simulink model "inverter_hil"  (R2024b)
settings: Solver=FixedStepDiscrete  StartTime=0.0  StopTime=inf  FixedStep=0.001  RelTol=1e-3
InitFcn:
  | inverterhil.enforceHardwarePreflight(bdroot);
values from neighbouring files (symbols this model uses):
  hil_cal_pedals_pressed_v1 = 1.1631952391851683    [inverter_hil.sldd]
  hil_cal_pedals_pressed_v2 = 2.341496910048066    [inverter_hil.sldd]
  hil_cal_pedals_pressed_v3 = 1.6012817578393226    [inverter_hil.sldd]
  hil_cal_pedals_pressed_v4 = 1.6012817578393226    [inverter_hil.sldd]
  hil_cal_pedals_released_v1 = 1.5156786449988555    [inverter_hil.sldd]
  hil_cal_pedals_released_v2 = 3.2025635156786452    [inverter_hil.sldd]
  hil_cal_pedals_released_v3 = 0.45445181963836118    [inverter_hil.sldd]
  hil_cal_pedals_released_v4 = 0.45445181963836118    [inverter_hil.sldd]
  hil_cmd_can_drop_control_mask = 0    [inverter_hil.sldd]
  hil_cmd_can_drop_status_mask = 0    [inverter_hil.sldd]
  hil_cmd_dc_link12_v = 0.0    [inverter_hil.sldd]
  hil_cmd_dc_link34_v = 0.0    [inverter_hil.sldd]
  hil_cmd_digital_cooling_switch = 0    [inverter_hil.sldd]
  hil_cmd_digital_main_button = 0    [inverter_hil.sldd]
  hil_cmd_digital_main_button_sequence = 0    [inverter_hil.sldd]
  hil_cmd_digital_precharge_sequence = 0    [inverter_hil.sldd]
  hil_cmd_digital_shutdown_feedback = 0    [inverter_hil.sldd]
  hil_cmd_gui_heartbeat = 0    [inverter_hil.sldd]
  hil_cmd_inverter1_connected = 1    [inverter_hil.sldd]
  hil_cmd_inverter1_fault_mask = 0    [inverter_hil.sldd]
  hil_cmd_inverter1_load_nm = 0.0    [inverter_hil.sldd]
  hil_cmd_inverter2_connected = 1    [inverter_hil.sldd]
  hil_cmd_inverter2_fault_mask = 0    [inverter_hil.sldd]
  hil_cmd_inverter2_load_nm = 0.0    [inverter_hil.sldd]
  hil_cmd_inverter3_connected = 1    [inverter_hil.sldd]
  hil_cmd_inverter3_fault_mask = 0    [inverter_hil.sldd]
  hil_cmd_inverter3_load_nm = 0.0    [inverter_hil.sldd]
  hil_cmd_inverter4_connected = 1    [inverter_hil.sldd]
  hil_cmd_inverter4_fault_mask = 0    [inverter_hil.sldd]
  hil_cmd_inverter4_load_nm = 0.0    [inverter_hil.sldd]
  hil_cmd_pedals_brake = 0.0    [inverter_hil.sldd]
  hil_cmd_pedals_plausibility_override = 0    [inverter_hil.sldd]
  hil_cmd_pedals_throttle = 0.0    [inverter_hil.sldd]
undefined symbols (not defined in the file or in its folder): Pull, up
libraries: speedgoatlib_IO614 x18, canmsglib x14, speedgoatlib_IO183 x8
(part 2 of 2)

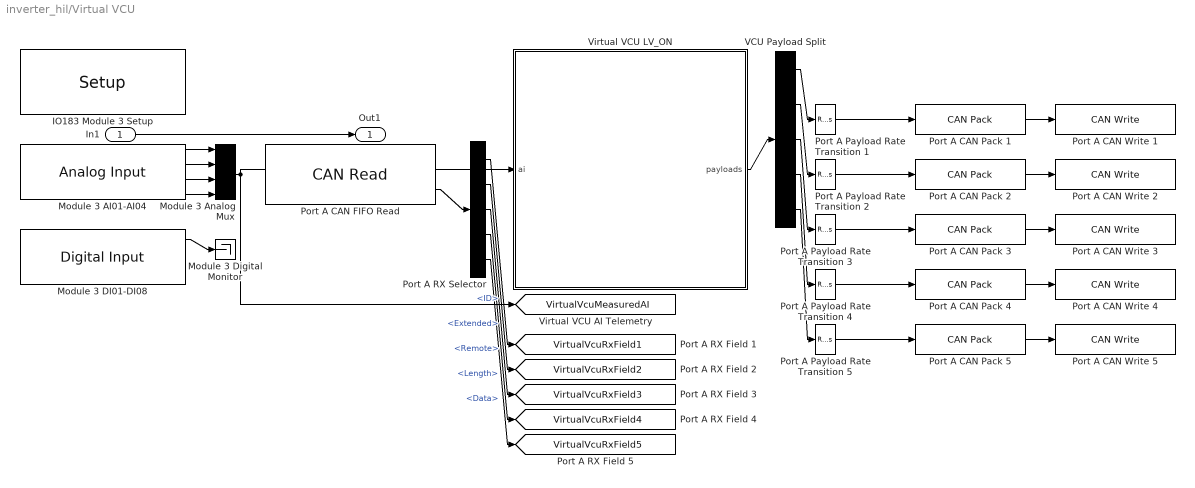
== system inverter_hil/Virtual VCU ==
  In1 : Inport
  IO183 Module 3 Setup : speedgoatlib_IO183/Setup  parModuleId=3  parPciSlot=-1  parDaSimult=on  parAdCoupling=Single Ended  parAdRange=0..5V  parAdChannelLow=1  parAdChannelHigh=4  parDaChannels=[1 2 3 4]  parDaRange=0..5V  parDaInit=[0 0 0 0]  parDaReset=[0 0 0 0]  parDoChannels=[1 2 3 4 5 6 7 8]  parDoInit=[0 0 0 0 0 0 0 0]  parDoReset=[0 0 0 0 0 0 0 0]  parDiChannels=[1 2 3 4 5 6 7 8]  parIOPullReferenceFront=Pull-down  parIOPullReferenceRear=Pull-up (3.3V)
      settings: SourceProductName=IO183
  Module 3 AI01-AI04 : speedgoatlib_IO183/Analog Input  Priority=0  parModuleId=3  parSampTime=0.001  parPciSlot=-1  parAdChannelLow=1  parAdChannelHigh=4
      settings: SourceProductName=IO183
  Module 3 Analog Mux : Mux
  Module 3 DI01-DI08 : speedgoatlib_IO183/Digital Input  parModuleId=3  parSampTime=0.001  parPciSlot=-1  parDiChannels=[1 2 3 4 5 6 7 8]
      settings: SourceProductName=IO183
  Module 3 Digital Monitor : Terminator
  Port A CAN FIFO Read : speedgoatlib_IO614/CAN Read   moduleType=IO614  id=1  channel=2  canType=CAN (HS)  useBusOut=on  HasMulRead=Single Read from Buffer (FIFO)  MsgIDlist=[1 2]  isEFF=off  LabelInHex=on  enableInput=off  ts=0.001  initValues=[614 1 0.001 1 1 1 0 1 0 1 2 1 2]
      settings: SourceProductName=IO614
  Port A CAN Pack 1 : canmsglib/CAN Pack  MsgList=(none)  MsgName=CAN Msg  MsgIDType=Standard (11-bit identifier)  MsgIdentifier=501  CANIDInput=off  MsgLength=8  Remote=off  ApplyMinMax=off  BusOutput=off  SignalInfo={}
      settings: LibrarySourceBlock=canlib/CAN Pack  DataFormat=raw data
  Port A CAN Pack 2 : canmsglib/CAN Pack  MsgList=(none)  MsgName=CAN Msg  MsgIDType=Standard (11-bit identifier)  MsgIdentifier=390  CANIDInput=off  MsgLength=8  Remote=off  ApplyMinMax=off  BusOutput=off  SignalInfo={}
      settings: LibrarySourceBlock=canlib/CAN Pack  DataFormat=raw data
  Port A CAN Pack 3 : canmsglib/CAN Pack  MsgList=(none)  MsgName=CAN Msg  MsgIDType=Standard (11-bit identifier)  MsgIdentifier=406  CANIDInput=off  MsgLength=8  Remote=off  ApplyMinMax=off  BusOutput=off  SignalInfo={}
      settings: LibrarySourceBlock=canlib/CAN Pack  DataFormat=raw data
  Port A CAN Pack 4 : canmsglib/CAN Pack  MsgList=(none)  MsgName=CAN Msg  MsgIDType=Standard (11-bit identifier)  MsgIdentifier=422  CANIDInput=off  MsgLength=8  Remote=off  ApplyMinMax=off  BusOutput=off  SignalInfo={}
      settings: LibrarySourceBlock=canlib/CAN Pack  DataFormat=raw data
  Port A CAN Pack 5 : canmsglib/CAN Pack  MsgList=(none)  MsgName=CAN Msg  MsgIDType=Standard (11-bit identifier)  MsgIdentifier=438  CANIDInput=off  MsgLength=8  Remote=off  ApplyMinMax=off  BusOutput=off  SignalInfo={}
      settings: LibrarySourceBlock=canlib/CAN Pack  DataFormat=raw data
  Port A CAN Write {1..5} (5 alike) : speedgoatlib_IO614/CAN Write   moduleType=IO614  id=1  channel=2  canType=CAN (HS)  useBusIn=off  numOfMsg=1  enableInput=off  enableStatusPort=on  initValues=[614 1 0.005 1 1 1 1 1 0 0]  ts=0.005
      settings: SourceProductName=IO614
  Port A Payload Rate Transition {1..5} (5 alike) : RateTransition
  Port A RX Selector : BusSelector  OutputSignals=ID,Extended,Remote,Length,Data
  VCU Payload Split : Demux  Outputs=[8 8 8 8 8]
  Virtual VCU LV_ON : MATLAB Function  TreatAsAtomicUnit=on
  Out1 : Outport
  tag scope: VirtualVcuMeasuredAI=global, VirtualVcuRxField1=global, VirtualVcuRxField2=global, VirtualVcuRxField3=global, VirtualVcuRxField4=global, VirtualVcuRxField5=global
  wires:
  In1/1 -> Out1/1
  Module 3 AI01-AI04/1 -> Module 3 Analog Mux/1
  Module 3 AI01-AI04/2 -> Module 3 Analog Mux/2
  Module 3 AI01-AI04/3 -> Module 3 Analog Mux/3
  Module 3 AI01-AI04/4 -> Module 3 Analog Mux/4
  Port A CAN FIFO Read/2 -> Port A RX Selector/1
  Module 3 Analog Mux/1 -> Virtual VCU LV_ON/1(ai), [VirtualVcuMeasuredAI]
  Virtual VCU LV_ON/1(payloads) -> VCU Payload Split/1
  Port A RX Selector/1 -> [VirtualVcuRxField1]  "<ID>"
  Port A RX Selector/2 -> [VirtualVcuRxField2]  "<Extended>"
  Port A RX Selector/3 -> [VirtualVcuRxField3]  "<Remote>"
  Port A RX Selector/4 -> [VirtualVcuRxField4]  "<Length>"
  Port A RX Selector/5 -> [VirtualVcuRxField5]  "<Data>"
  Module 3 DI01-DI08/1 -> Module 3 Digital Monitor/1
  VCU Payload Split/1 -> Port A Payload Rate Transition 1/1
  Port A Payload Rate Transition 1/1 -> Port A CAN Pack 1/1
  Port A CAN Pack 1/1 -> Port A CAN Write 1/1
  VCU Payload Split/2 -> Port A Payload Rate Transition 2/1
  Port A Payload Rate Transition 2/1 -> Port A CAN Pack 2/1
  Port A CAN Pack 2/1 -> Port A CAN Write 2/1
  VCU Payload Split/3 -> Port A Payload Rate Transition 3/1
  Port A Payload Rate Transition 3/1 -> Port A CAN Pack 3/1
  Port A CAN Pack 3/1 -> Port A CAN Write 3/1
  VCU Payload Split/4 -> Port A Payload Rate Transition 4/1
  Port A Payload Rate Transition 4/1 -> Port A CAN Pack 4/1
  Port A CAN Pack 4/1 -> Port A CAN Write 4/1
  VCU Payload Split/5 -> Port A Payload Rate Transition 5/1
  Port A Payload Rate Transition 5/1 -> Port A CAN Pack 5/1
  Port A CAN Pack 5/1 -> Port A CAN Write 5/1

== matlab function inverter_hil/Virtual VCU/Virtual VCU LV_ON ==
  data: ai input; payloads output
function payloads = virtualVcuDeployStep(ai)
%#codegen
payloads = zeros(40,1,'uint8');
t = uint8(max(0,min(100,round(ai(1) * 20))));
payloads(1) = t;
payloads(2) = uint8(max(0,min(255,round(ai(3) * 130))));
payloads(9) = 1; payloads(11) = 80; payloads(12) = 70;
payloads(17) = 1; payloads(19) = 80; payloads(20) = 70;
payloads(25) = 1; payloads(27) = 80; payloads(28) = 70;
payloads(33) = 1; payloads(35) = 80; payloads(36) = 70;
end

== matlab function inverter_hil/Hardware I O - PRE-FLIGHT DISABLED/Status Transmit Mask ==
  data: dropStatusMask input; k1 output; k2 output; k3 output; k4 output; k5 output; k6 output; k7 output; k8 output; k9 output
function [k1,k2,k3,k4,k5,k6,k7,k8,k9] = ...
    ephorusStatusTransmitMask(dropStatusMask)
%#codegen
%EPHORUSSTATUSTRANSMITMASK Fix 4: split INVERTERHIL.STATUSTRANSMITMASK's
%9-entry keep vector into nine scalar Tx Control outputs, one per
%CAN Write block in INVERTERHIL.PROTOCOL status-cycle order, because
%each CAN Write's Tx Control port takes a scalar and a MATLAB
%Function block cannot emit a bus without a Simulink.Bus definition.
%
%CAN Write's Tx Control input is uint32 (a transmit-count control, not
%a boolean enable), so KEEP is cast rather than passed as logical: 1 to
%transmit this tick, 0 to genuinely skip it.
keep = uint32(inverterhil.statusTransmitMask(dropStatusMask));
k1 = keep(1); k2 = keep(2); k3 = keep(3);
k4 = keep(4); k5 = keep(5); k6 = keep(6);
k7 = keep(7); k8 = keep(8); k9 = keep(9);
end

== matlab function inverter_hil/Ephorus System Status/Ephorus Status Cycle ==
  data: rxDataPresent input; payloads output; rxId input; rxExtended input; rxRemote input; rxLength input; rxData input; loadNm1 input; loadNm2 input; loadNm3 input; loadNm4 input; connected1 input; connected2 input; connected3 input; connected4 input; dcLink12V input; dcLink34V input; dropControlMask input; rxObservation output
function [payloads, rxObservation] = ephorusSystemStatusStep( ...
    rxDataPresent, rxId, rxExtended, rxRemote, rxLength, rxData, ...
    loadNm1, loadNm2, loadNm3, loadNm4, ...
    connected1, connected2, connected3, connected4, ...
    dcLink12V, dcLink34V, dropControlMask)
%#codegen
%EPHORUSSYSTEMSTATUSSTEP Advance the real, persistent-state Ephorus
%status cycle (see INVERTERHIL.STEPMODEL) and emit its nine 8-byte
%payloads. Single source of truth: the hardware boundary reads this
%same signal through a Goto/From pair rather than recomputing it.
%
%The RX inputs are one received CAN frame per step, published by the
%hardware boundary. BANK is persistent so a retained command survives
%across ticks, which is what lets a commanding VCU move a channel out
%of Idle.
%
%A frame is ALWAYS passed, with DROP set when nothing was received.
%RECEIVECONTROLFRAME rejects a dropped frame without touching the
%bank, so the array stays fixed-size for code generation instead of
%growing and shrinking. Nothing is fabricated: no data present means
%no command retained, exactly as before this input existed.
%
%LOADNM1-4, CONNECTED1-4, DCLINK12V/34V and DROPCONTROLMASK are GUI
%COMMAND PARAMETERS' Gotos (Fix 2, Fix 4), read here rather than by
%recomputing anything the dead "Ephorus Channel 1-4" scaffold would
%have provided.
persistent state plantState tickMs bank statusBank
if isempty(state)
    state = inverterhil.initialSystemState();
    plantState = inverterhil.initialPlantState();
    tickMs = uint32(0);
    bank = inverterhil.initialDecoderBank();
    statusBank = inverterhil.initialStatusBank();
end
%(:)' normalises the bus Data element to a 1x8 row regardless of the
%orientation Simulink propagates, matching the proven pattern in the
%IO614 CAN visibility test decoder.
payload = uint8(rxData(:))';
frame = struct( ...
    'id', uint32(rxId), ...
    'dlc', uint8(rxLength), ...
    'payload', payload, ...
    'isExtended', logical(rxExtended), ...
    'isRemote', logical(rxRemote), ...
    'drop', ~logical(rxDataPresent));
%CONFIG and CAL are passed explicitly rather than as [] so the
%variable never changes type: code generation rejects a double []
%being reassigned to a struct inside STEPMODEL's defaulting branch.
    statusBank = inverterhil.receiveStatusFrame(statusBank, frame, tickMs);
%EXTERNALINPUTS carries the GUI-commanded per-channel load torque, DC
%link pair voltage (dcLink12V feeds channels 1-2, dcLink34V feeds
%channels 3-4, matching ADDARCHITECTURE's dcPort = 1 + (channel > 2)
%convention), and connected flag into STEPMODEL -- see
%INVERTERHIL.DEFAULTEXTERNALINPUTS for why faultMask is left at its
%default (no consumer exists for it yet).
externalInputs = inverterhil.defaultExternalInputs();
externalInputs.channels(1).loadTorqueNm = double(loadNm1);
externalInputs.channels(2).loadTorqueNm = double(loadNm2);
externalInputs.channels(3).loadTorqueNm = double(loadNm3);
externalInputs.channels(4).loadTorqueNm = double(loadNm4);
externalInputs.channels(1).connected = logical(connected1);
externalInputs.channels(2).connected = logical(connected2);
externalInputs.channels(3).connected = logical(connected3);
externalInputs.channels(4).connected = logical(connected4);
externalInputs.channels(1).dcLinkV = double(dcLink12V);
externalInputs.channels(2).dcLinkV = double(dcLink12V);
externalInputs.channels(3).dcLinkV = double(dcLink34V);
externalInputs.channels(4).dcLinkV = double(dcLink34V);
%The CAN control-frame drop mask (Fix 4) is applied to a COPY of the
%received frame used only for retention -- STATUSBANK above already
%saw the unmodified FRAME, so this mask cannot affect the received-
%status-frame path, only whether a control frame is retained into the
%decoder bank.
controlFrame = inverterhil.applyControlDropMask(frame, uint8(dropControlMask));
[state, plantState, cycle, ~, ~, bank] = inverterhil.stepModel( ...
    state, plantState, tickMs, inverterhil.defaultStateConfig(), ...
    inverterhil.defaultCalibration(), bank, controlFrame, ...
    externalInputs);
%RXOBSERVATION is taken BEFORE the tick advances, so the ages it
%reports are measured against the same tick the frame above was
%retained at. Advancing first would make a frame received this step
%appear one period old.
controlRows = inverterhil.rxObservation(bank, tickMs);
statusRows = inverterhil.statusObservation(statusBank, tickMs);
rxObservation = zeros(13, 14);
rxObservation(1:4, :) = controlRows;
rxObservation(5:13, 1:11) = statusRows;
%TICKMS is REAL MILLISECONDS, so it must advance by this block's
%period (5 ms), not by 1. It previously incremented by 1 per
%execution while DECODERSNAPSHOT compared the resulting age against
%PROTOCOL.TIMING.COMMANDTORQUEZEROMS (50) and COMMANDERRORMS (500),
%which are genuine millisecond thresholds. At a 5 ms period that
%made every command timeout 5x too slow: torque zeroed at 250 ms
%instead of 50, and Error latched at 2500 ms instead of 500. A rig
%that reports a VCU meeting a watchdog deadline it actually misses
%is worse than no rig, so this is derived from the same constant
%that sets the block sample time rather than written as a literal.
%
%The MOD wrap is also deliberate. MATLAB uint32 addition SATURATES,
%and the generated C++ made that explicit:
%    if (t + 1U < t) { t = MAX_uint32_T; }
%so the counter would FREEZE at intmax rather than roll over. Once
%frozen every newly retained frame reads age 0 forever and command
%timeouts stop firing entirely. DECODERSNAPSHOT already measures
%ages with modulo arithmetic, so a true wrap is what it expects.
tickMs = uint32(mod(double(tickMs) + 5, 4294967296));
payloads = cycle.payloads;
end

== matlab function inverter_hil/Hardware I O - PRE-FLIGHT DISABLED/Ephorus Status Cycle Frames ==
  data: payloads input; f1 output; f2 output; f3 output; f4 output; f5 output; f6 output; f7 output; f8 output; f9 output
function [f1,f2,f3,f4,f5,f6,f7,f8,f9] = ephorusStatusCycleFrames(payloads)
%EPHORUSSTATUSCYCLEFRAMES Split the nine-frame status cycle into the
%nine 1x8 rows the CAN Pack blocks need, one per status ID, in the
%order INVERTERHIL.PROTOCOL declares.
f1 = payloads(1,:); f2 = payloads(2,:); f3 = payloads(3,:);
f4 = payloads(4,:); f5 = payloads(5,:); f6 = payloads(6,:);
f7 = payloads(7,:); f8 = payloads(8,:); f9 = payloads(9,:);
end

== matlab function inverter_hil/Hardware I O - PRE-FLIGHT DISABLED/Pedal Voltage Calibration ==
  data: throttle input; ao1 output; brake input; released1 input; pressed1 input; released2 input; pressed2 input; released3 input; pressed3 input; released4 input; pressed4 input; ao2 output; ao3 output; ao4 output
function [ao1,ao2,ao3,ao4] = pedalVoltageCalibration( ...
    throttle, brake, released1, pressed1, released2, pressed2, ...
    released3, pressed3, released4, pressed4)
%PEDALVOLTAGECALIBRATION Map GUI throttle/brake fractions (0-1) to
%the four redundant IO183 analog-output voltages using the
%calibrated released/pressed endpoints.
%
%   HIL_CAL_PEDALS_RELEASED_V*/PRESSED_V* ship as NaN precisely so an
%   uncalibrated channel is detectable rather than silently plausible
%   (INVERTER_HIL_PLAN.MD S3.1 requires each endpoint be measured at
%   the connected VCU pin under load). An uncalibrated or out-of-range
%   channel therefore drives 0 V -- the same level the IO183 initial
%   and reset values use -- instead of propagating NaN into a DAC.
ao1 = calibratedVolts(released1, pressed1, throttle);
ao2 = calibratedVolts(released2, pressed2, throttle);
ao3 = calibratedVolts(released3, pressed3, brake);
ao4 = calibratedVolts(released4, pressed4, brake);
end

function volts = calibratedVolts(releasedV, pressedV, fraction)
if ~isfinite(releasedV) || ~isfinite(pressedV) || ~isfinite(fraction)
    volts = 0;
    return
end
bounded = min(max(fraction, 0), 1);
volts = releasedV + (pressedV - releasedV) * bounded;
%The IO183 analog outputs are configured for the 0..5 V range.
volts = min(max(volts, 0), 5);
end

== matlab function inverter_hil/Hardware I O - PRE-FLIGHT DISABLED/Precharge Pulse Generator ==
  data: counter input; active output
function active = prechargePulseFromCounter(counter)
%PRECHARGEPULSEFROMCOUNTER Turn a GUI counter increment into a
%fixed-width PRECH_BTN_IN pulse (INVERTER_HIL_PLAN.MD S7.1: "Model
%generates a deterministic precharge pulse on counter change").
%200 ms (at the model's 1 ms base rate) is provisional pending
%confirmation against VCU firmware precharge-button timing.
persistent prevCounter ticksRemaining initialized
pulseTicks = uint32(200);
if isempty(initialized)
    prevCounter = counter;
    ticksRemaining = uint32(0);
    initialized = true;
end
if counter ~= prevCounter
    ticksRemaining = pulseTicks;
    prevCounter = counter;
end
%Emitted as double because that is what the IO183 Digital Output
%port takes.
active = double(ticksRemaining > uint32(0));
if ticksRemaining > uint32(0)
    ticksRemaining = ticksRemaining - uint32(1);
end
end
